simulink subsystem "PvtSubSys_LATC"  (R2020b)
settings: Solver=VariableStepAuto  StartTime=0.0  StopTime=10.0  RelTol=1e-3
values from neighbouring files (symbols this model uses):
  P_Global_CharSpd_ms : value not decoded    [PubParsGlobal.sldd]
  P_Global_SteeringAngleRatio : value not decoded    [PubParsGlobal.sldd]
  P_Global_WheelBase_m : value not decoded    [PubParsGlobal.sldd]
  P_LCS_A0_Limit = 0.25    [LATC.sldd]    (also in LCS_v05.sldd)
  P_LCS_A1_Limit = 0.002    [LATC.sldd]    (also in LCS_v05.sldd)
  P_LCS_communicationTest = 1.0    [LATC.sldd]    (also in LCS_v05.sldd)
  P_LCS_Current_Offset_Test_SW = 0.0    [LATC.sldd]
  P_LCS_Current_Offset_Test_Value = 0.0    [LATC.sldd]
  P_LCS_Curvature_bp : value not decoded    [LATC.sldd]
  P_LCS_CycleTime = 0.4 0.4 0.4 0.4 0.4 0.4 0.4 0.4 0.4 0.6 0.6 0.6 0.6 0.6 0.6 0.6 0.4 0.4 0.4 0.4 0.4 0.4 0.4 0.4 0.4 0.6 0.6 0.6 0.6 0.6 0.6 0.6 0.4 0.4 0.4 0.4 0.4 0.4 0.4 0.4 0.4 0.6 0.6 0.6 0.6 0.6 0.6 0.6 0.4 0.4 0.4 0.4 0.4 0.4 0.4 0.4 0.4 0.6 0.6 0.6 0.6 0.6 0.6 0.6 0.4 0.4 0.4 0.4 0.4 0.4 0.4 0.4 0.4 0.6 0.6 0.6 0.6 0.6 0.6 0.6 0.4 0.4 0.4 0.4 0.4 0.4 0.4 0.4 0.4 0.6 0.6 0.6 0.6 0.6 0.6 0.6 0.4 0.4 0.4 0.4    [LATC.sldd]
  P_LCS_ESS_AngleSlope_Limit = 2.9    [LATC.sldd]    (also in LCS_v05.sldd)
  P_LCS_IN_Offset_Test_SW = 0.0    [LATC.sldd]    (also in LCS_v05.sldd)
  P_LCS_IN_Offset_Test_Value = 0.0    [LATC.sldd]    (also in LCS_v05.sldd)
  P_LCS_LATC_CurOffsetVehicleSpdLimitValue_degs = 7.0    [LATC.sldd]
  P_LCS_LATC_Du_Max = 20.0    [LATC.sldd]
  P_LCS_LATC_ELKAngleSlope_ratio : value not decoded    [LATC.sldd]
  P_LCS_LATC_ELKMaxLatAcc_ms2 : value not decoded    [LATC.sldd]
  P_LCS_LATC_ESSAngleSlope_ratio : value not decoded    [LATC.sldd]
  P_LCS_LATC_ESSMaxLatAcc_ms2 : value not decoded    [LATC.sldd]
  P_LCS_LATC_LCAngleSlope_ratio : value not decoded    [LATC.sldd]
  P_LCS_LATC_LCCancleMaxLatAcc_ms2 : value not decoded    [LATC.sldd]
  P_LCS_LATC_LCEcoAngleSlope_ratio : value not decoded    [LATC.sldd]
  P_LCS_LATC_LCEcoMaxLatAcc_ms2 : value not decoded    [LATC.sldd]
  P_LCS_LATC_LCKAngleSlope_ratio : value not decoded    [LATC.sldd]
  P_LCS_LATC_LCKIEAngleSlope_ratio : value not decoded    [LATC.sldd]
  P_LCS_LATC_LCKIEMaxLatAcc_ms2 : value not decoded    [LATC.sldd]
  P_LCS_LATC_LCKMaxLatAcc_ms2 : value not decoded    [LATC.sldd]
  P_LCS_LATC_LCNormalAngleSlope_ratio : value not decoded    [LATC.sldd]
  P_LCS_LATC_LCNormalMaxLatAcc_ms2 : value not decoded    [LATC.sldd]
  P_LCS_LATC_LCSportAngleSlope_ratio : value not decoded    [LATC.sldd]
  P_LCS_LATC_LCSportMaxLatAcc_ms2 : value not decoded    [LATC.sldd]
  P_LCS_LATC_LKAAngleSlope_ratio : value not decoded    [LATC.sldd]
  P_LCS_LATC_LKAMaxLatAcc_ms2 : value not decoded    [LATC.sldd]
  P_LCS_LATC_MatrixQ1_st = 0.8 0.8 1.2 1.4 1.4 1.4 2.0 2.2 2.2 2.2 2.2 2.2 2.2 2.2 2.2 2.2 0.8 0.8 1.2 1.4 1.4 1.4 2.0 2.2 2.2 2.2 2.2 2.2 2.2 2.2 2.2 2.2 0.8 0.8 1.2 1.4 1.4 1.4 2.0 2.2 2.2 2.2 2.2 2.2 2.2 2.2 2.2 2.2 0.8 0.8 1.2 1.4 1.4 1.4 2.0 2.2 2.2 2.2 2.2 2.2 2.2 2.2 2.2 2.2 0.8 0.8 1.2 1.4 1.4 1.4 2.0 2.2 2.2 2.2 2.2 2.2 2.2 2.2 2.2 2.2 0.8 0.8 1.2 1.4 1.4 1.4 2.0 2.2 2.2 2.2 2.2 2.2 2.2 2.2 2.2 2.2 0.8 0.8 1.2 1.4    [LATC.sldd]
  P_LCS_LATC_MatrixQ3_st = 20.0 20.0 20.0 20.0 20.0 15.0 15.0 15.0 15.0 15.0 15.0 15.0 15.0 13.0 13.0 13.0 20.0 20.0 20.0 20.0 20.0 15.0 15.0 15.0 15.0 15.0 15.0 15.0 15.0 13.0 13.0 13.0 20.0 20.0 20.0 20.0 20.0 15.0 15.0 15.0 15.0 15.0 15.0 15.0 15.0 13.0 13.0 13.0 20.0 20.0 20.0 20.0 20.0 15.0 15.0 15.0 15.0 15.0 15.0 15.0 15.0 13.0 13.0 13.0 20.0 20.0 20.0 20.0 20.0 15.0 15.0 15.0 15.0 15.0 15.0 15.0 15.0 13.0 13.0 13.0    [LATC.sldd]
  P_LCS_LATC_MatrixR_st = 10.0 10.0 10.0 10.0 10.0 10.0 10.0 15.0 15.0 15.0 15.0 15.0 15.0 15.0 15.0 15.0 10.0 10.0 10.0 10.0 10.0 10.0 10.0 15.0 15.0 15.0 15.0 15.0 15.0 15.0 15.0 15.0 10.0 10.0 10.0 10.0 10.0 10.0 10.0 15.0 15.0 15.0 15.0 15.0 15.0 15.0 15.0 15.0 10.0 10.0 10.0 10.0 10.0 10.0 10.0 15.0 15.0 15.0 15.0 15.0 15.0 15.0 15.0 15.0 10.0 10.0 10.0 10.0 10.0 10.0 10.0 15.0 15.0 15.0 15.0 15.0 15.0 15.0 15.0 15.0    [LATC.sldd]
  P_LCS_LATC_Max_LatAcc = 4.0    [LATC.sldd]
  P_LCS_LATC_Max_Phi = 15.0    [LATC.sldd]
  P_LCS_LATC_Max_y = 0.5    [LATC.sldd]
  P_LCS_LATC_MPC_SW = 0.0    [LATC.sldd]
  P_LCS_LATC_PreView_SW = 1.0    [LATC.sldd]
  P_LCS_LATC_SoftConstWeight = 1.0    [LATC.sldd]
  P_LCS_LATC_StateActivAngleSlopeLimit_ratio : value not decoded    [LATC.sldd]
  P_LCS_LATC_StateActiveFlg_TabX_st : value not decoded    [LATC.sldd]
  P_LCS_LATC_StateActiveHoldTime_TabY_st : value not decoded    [LATC.sldd]
  P_LCS_LATC_StateHoldTime_st = 250.0    [LATC.sldd]
  P_LCS_LATC_TarAngleFliterWindowSize = 5.0    [LATC.sldd]
  P_LCS_LATC_TarAngleLP_Time = 0.02    [LATC.sldd]
  P_LCS_LATC_U_Max = 90.0    [LATC.sldd]
  P_LCS_LCK_AngleSlope_Limit = 1.4    [LATC.sldd]
  P_LCS_LineVaildSW = 0.0    [LATC.sldd]
  P_LCS_Lookahead_Distance : value not decoded    [LATC.sldd]
  P_LCS_Lookahead_DistanceFac : value not decoded    [LATC.sldd]
  P_LCS_PLAN_CurvePreView_s = 0.3    [LATC.sldd]
  P_LCS_PLAN_CurvePreview_TabX_m : value not decoded    [LATC.sldd]
  P_LCS_PLAN_CurvePreViewFilterTime_s = 0.1    [LATC.sldd]
  P_LCS_PLAN_ELKAyDtLimit_Tab_ms3 = 1.0 1.0 1.0 1.0 1.0 1.0 1.0 1.0 1.0 1.0 1.0 1.0 1.0 1.0 1.0 1.0 1.0 1.0 1.0 1.0 1.0 1.0 1.0 1.0 1.0 1.0 1.0 1.0 1.0 1.0 1.0 1.0 1.0 1.0 1.0 1.0 1.0 1.0 1.0 1.0 1.0 1.0 1.0 1.0 1.0 1.0 1.0 1.0 1.0 1.0 1.0 1.0 1.0 1.0 1.0 1.0 1.0 1.0 1.0 1.0 1.0 1.0 1.0 1.0 1.0 1.0 1.0 1.0 1.0 1.0 1.0 1.0 1.0 1.0 1.0 1.0 1.0 1.0 1.0 1.0 1.0 1.0 1.0 1.0 1.0 1.0 1.0 1.0 1.0 1.0 1.0 1.0 1.0 1.0 1.0 1.0 1.0 1.0 1.0 1.0    [LATC.sldd]
  P_LCS_PLAN_ESSAyDtLimit_Tab_ms3 = 1.0 1.0 1.0 1.0 1.0 1.0 1.0 1.0 1.0 1.0 1.0 1.0 1.0 1.0 1.0 1.0 1.0 1.0 1.0 1.0 1.0 1.0 1.0 1.0 1.0 1.0 1.0 1.0 1.0 1.0 1.0 1.0 1.0 1.0 1.0 1.0 1.0 1.0 1.0 1.0 1.0 1.0 1.0 1.0 1.0 1.0 1.0 1.0 1.0 1.0 1.0 1.0 1.0 1.0 1.0 1.0 1.0 1.0 1.0 1.0 1.0 1.0 1.0 1.0 1.0 1.0 1.0 1.0 1.0 1.0 1.0 1.0 1.0 1.0 1.0 1.0 1.0 1.0 1.0 1.0 1.0 1.0 1.0 1.0 1.0 1.0 1.0 1.0 1.0 1.0 1.0 1.0 1.0 1.0 1.0 1.0 1.0 1.0 1.0 1.0    [LATC.sldd]
  P_LCS_PLAN_LCCancleAyDtLimit_Tab_ms3 = 1.0 1.0 1.0 1.0 1.0 1.0 1.0 1.0 1.0 1.0 1.0 1.0 1.0 1.0 1.0 1.0 1.0 1.0 1.0 1.0 1.0 1.0 1.0 1.0 1.0 1.0 1.0 1.0 1.0 1.0 1.0 1.0 1.0 1.0 1.0 1.0 1.0 1.0 1.0 1.0 1.0 1.0 1.0 1.0 1.0 1.0 1.0 1.0 1.0 1.0 1.0 1.0 1.0 1.0 1.0 1.0 1.0 1.0 1.0 1.0 1.0 1.0 1.0 1.0 1.0 1.0 1.0 1.0 1.0 1.0 1.0 1.0 1.0 1.0 1.0 1.0 1.0 1.0 1.0 1.0 1.0 1.0 1.0 1.0 1.0 1.0 1.0 1.0 1.0 1.0 1.0 1.0 1.0 1.0 1.0 1.0 1.0 1.0 1.0 1.0    [LATC.sldd]
  P_LCS_PLAN_LCEcoAyDtLimit_Tab_ms3 = 1.0 1.0 1.0 1.0 1.0 1.0 1.0 1.0 1.0 1.0 1.0 1.0 1.0 1.0 1.0 1.0 1.0 1.0 1.0 1.0 1.0 1.0 1.0 1.0 1.0 1.0 1.0 1.0 1.0 1.0 1.0 1.0 1.0 1.0 1.0 1.0 1.0 1.0 1.0 1.0 1.0 1.0 1.0 1.0 1.0 1.0 1.0 1.0 1.0 1.0 1.0 1.0 1.0 1.0 1.0 1.0 1.0 1.0 1.0 1.0 1.0 1.0 1.0 1.0 1.0 1.0 1.0 1.0 1.0 1.0 1.0 1.0 1.0 1.0 1.0 1.0 1.0 1.0 1.0 1.0 1.0 1.0 1.0 1.0 1.0 1.0 1.0 1.0 1.0 1.0 1.0 1.0 1.0 1.0 1.0 1.0 1.0 1.0 1.0 1.0    [LATC.sldd]
  P_LCS_PLAN_LCKAyDtLimit_Tab_ms3 = 1.5 1.5 1.5 1.5 1.5 1.5 1.5 1.5 1.5 1.5 1.5 1.5 1.5 1.5 1.5 1.5 1.5 1.5 1.5 1.5 1.5 1.5 1.5 1.5 1.5 1.5 1.5 1.5 1.5 1.5 1.5 1.5 1.5 1.5 1.5 1.5 1.5 1.5 1.5 1.5 1.5 1.5 1.5 1.5 1.5 1.5 1.5 1.5 1.5 1.5 1.5 1.5 1.5 1.5 1.5 1.5 1.5 1.5 1.5 1.5 1.5 1.5 1.5 1.5 1.5 1.5 1.5 1.5 1.5 1.5 1.5 1.5 1.5 1.5 1.5 1.5 1.5 1.5 1.5 1.5 1.5 1.5 1.5 1.5 1.5 1.5 1.5 1.5 1.5 1.5 1.5 1.5 1.5 1.5 1.5 1.5 1.5 1.5 1.5 1.5    [LATC.sldd]
  P_LCS_PLAN_LCKIEAyDtLimit_Tab_ms3 = 1.0 1.0 1.0 1.0 1.0 1.0 1.0 1.0 1.0 1.0 1.0 1.0 1.0 1.0 1.0 1.0 1.0 1.0 1.0 1.0 1.0 1.0 1.0 1.0 1.0 1.0 1.0 1.0 1.0 1.0 1.0 1.0 1.0 1.0 1.0 1.0 1.0 1.0 1.0 1.0 1.0 1.0 1.0 1.0 1.0 1.0 1.0 1.0 1.0 1.0 1.0 1.0 1.0 1.0 1.0 1.0 1.0 1.0 1.0 1.0 1.0 1.0 1.0 1.0 1.0 1.0 1.0 1.0 1.0 1.0 1.0 1.0 1.0 1.0 1.0 1.0 1.0 1.0 1.0 1.0 1.0 1.0 1.0 1.0 1.0 1.0 1.0 1.0 1.0 1.0 1.0 1.0 1.0 1.0 1.0 1.0 1.0 1.0 1.0 1.0    [LATC.sldd]
  P_LCS_PLAN_LCNormalAyDtLimit_Tab_ms3 = 1.0 1.0 1.0 1.0 1.0 1.0 1.0 1.0 1.0 1.0 1.0 1.0 1.0 1.0 1.0 1.0 1.0 1.0 1.0 1.0 1.0 1.0 1.0 1.0 1.0 1.0 1.0 1.0 1.0 1.0 1.0 1.0 1.0 1.0 1.0 1.0 1.0 1.0 1.0 1.0 1.0 1.0 1.0 1.0 1.0 1.0 1.0 1.0 1.0 1.0 1.0 1.0 1.0 1.0 1.0 1.0 1.0 1.0 1.0 1.0 1.0 1.0 1.0 1.0 1.0 1.0 1.0 1.0 1.0 1.0 1.0 1.0 1.0 1.0 1.0 1.0 1.0 1.0 1.0 1.0 1.0 1.0 1.0 1.0 1.0 1.0 1.0 1.0 1.0 1.0 1.0 1.0 1.0 1.0 1.0 1.0 1.0 1.0 1.0 1.0    [LATC.sldd]
  P_LCS_PLAN_LCSportAyDtLimit_Tab_ms3 = 1.0 1.0 1.0 1.0 1.0 1.0 1.0 1.0 1.0 1.0 1.0 1.0 1.0 1.0 1.0 1.0 1.0 1.0 1.0 1.0 1.0 1.0 1.0 1.0 1.0 1.0 1.0 1.0 1.0 1.0 1.0 1.0 1.0 1.0 1.0 1.0 1.0 1.0 1.0 1.0 1.0 1.0 1.0 1.0 1.0 1.0 1.0 1.0 1.0 1.0 1.0 1.0 1.0 1.0 1.0 1.0 1.0 1.0 1.0 1.0 1.0 1.0 1.0 1.0 1.0 1.0 1.0 1.0 1.0 1.0 1.0 1.0 1.0 1.0 1.0 1.0 1.0 1.0 1.0 1.0 1.0 1.0 1.0 1.0 1.0 1.0 1.0 1.0 1.0 1.0 1.0 1.0 1.0 1.0 1.0 1.0 1.0 1.0 1.0 1.0    [LATC.sldd]
  P_LCS_PLAN_LKAAyDtLimit_Tab_ms3 = 1.0 1.0 1.0 1.0 1.0 1.0 1.0 1.0 1.0 1.0 1.0 1.0 1.0 1.0 1.0 1.0 1.0 1.0 1.0 1.0 1.0 1.0 1.0 1.0 1.0 1.0 1.0 1.0 1.0 1.0 1.0 1.0 1.0 1.0 1.0 1.0 1.0 1.0 1.0 1.0 1.0 1.0 1.0 1.0 1.0 1.0 1.0 1.0 1.0 1.0 1.0 1.0 1.0 1.0 1.0 1.0 1.0 1.0 1.0 1.0 1.0 1.0 1.0 1.0 1.0 1.0 1.0 1.0 1.0 1.0 1.0 1.0 1.0 1.0 1.0 1.0 1.0 1.0 1.0 1.0 1.0 1.0 1.0 1.0 1.0 1.0 1.0 1.0 1.0 1.0 1.0 1.0 1.0 1.0 1.0 1.0 1.0 1.0 1.0 1.0    [LATC.sldd]
  P_LCS_PLAN_MinPlanDis_m : value not decoded    [LATC.sldd]
  P_LCS_PLAN_PreCurMinDisFac_ratio : value not decoded    [LATC.sldd]
  P_LCS_PLAN_PreDisCurve_TabX_m : value not decoded    [LATC.sldd]
  P_LCS_PLAN_StateActiv_AyDtLimit_ms3 : value not decoded    [LATC.sldd]
  P_LCS_PLAN_VehicleSpd_TabX_kph : value not decoded    [LATC.sldd]
  P_LCS_PLAN_VehicleSpd_TabY_Kph : value not decoded    [LATC.sldd]
  P_LCS_Trq_Switch = 0.0    [LATC.sldd]    (also in LCS_v05.sldd)
  P_LCS_VehicleSpd_TabX_Kph : value not decoded    [LATC.sldd]
undefined symbols (not defined in the file or in its folder): HWP_AngCmdReqVal, HWP_AngCmdReqValVld, HWP_FuncTrqCmdReqFlag, HWP_ReqCtrlEPS, HWP_ReqCtrlEPSVld, HWP_TrqOvlCmdReqValue, HWP_WorkReq, HWP_WorkReqVld
libraries: simulink x4, dspbuff3 x2
(part 5 of 8)

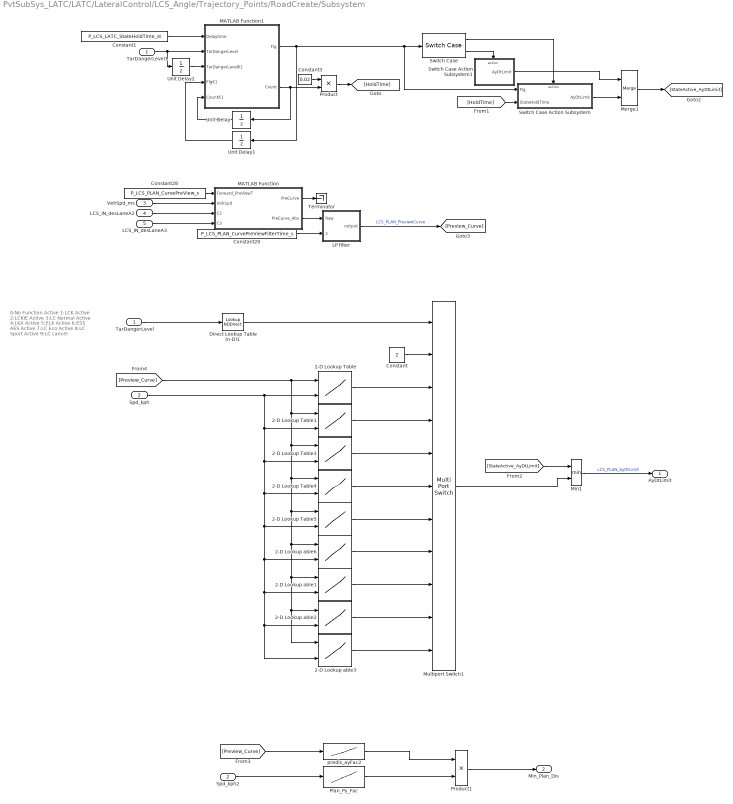
== system PvtSubSys_LATC/LATC/LateralControl/LCS_Angle/Trajectory_Points/RoadCreate/Subsystem ==
  note: 0:No Function Active
      | 1:LCK Active
      | 2:LCKIE Active
      | 3:LC Normal Active
      | 4:LKA Active
      | 5:ELK Active
      | 6:ESS AES Active
      | 7:LC Eco Active
      | 8:LC Sport Active
      | 9:LC cancel
  TarDangerLevel : Inport
  Spd_kph : Inport  Port=2
  VehSpd_ms : Inport  Port=3
  LCS_IN_desLaneA2 : Inport  Port=4
  LCS_IN_desLaneA3 : Inport  Port=5
  2-D Lookup Table : Lookup_n-D  BreakpointsForDimension1=P_LCS_PLAN_PreDisCurve_TabX_m  BreakpointsForDimension2=P_LCS_PLAN_VehicleSpd_TabY_Kph  Table=P_LCS_PLAN_LCKAyDtLimit_Tab_ms3  InternalRulePriority=Speed  RndMeth=Simplest  InputSameDT=on
      settings: InputPortMap=u0,u1
  2-D Lookup Table1 : Lookup_n-D  BreakpointsForDimension1=P_LCS_PLAN_PreDisCurve_TabX_m  BreakpointsForDimension2=P_LCS_PLAN_VehicleSpd_TabY_Kph  Table=P_LCS_PLAN_LCKIEAyDtLimit_Tab_ms3  InternalRulePriority=Speed  RndMeth=Simplest  InputSameDT=on
      settings: InputPortMap=u0,u1
  2-D Lookup Table3 : Lookup_n-D  BreakpointsForDimension1=P_LCS_PLAN_PreDisCurve_TabX_m  BreakpointsForDimension2=P_LCS_PLAN_VehicleSpd_TabY_Kph  Table=P_LCS_PLAN_LCNormalAyDtLimit_Tab_ms3  InternalRulePriority=Speed  RndMeth=Simplest  InputSameDT=on
      settings: InputPortMap=u0,u1
  2-D Lookup Table4 : Lookup_n-D  BreakpointsForDimension1=P_LCS_PLAN_PreDisCurve_TabX_m  BreakpointsForDimension2=P_LCS_PLAN_VehicleSpd_TabY_Kph  Table=P_LCS_PLAN_LKAAyDtLimit_Tab_ms3  InternalRulePriority=Speed  RndMeth=Simplest  InputSameDT=on
      settings: InputPortMap=u0,u1
  2-D Lookup Table5 : Lookup_n-D  BreakpointsForDimension1=P_LCS_PLAN_PreDisCurve_TabX_m  BreakpointsForDimension2=P_LCS_PLAN_VehicleSpd_TabY_Kph  Table=P_LCS_PLAN_ELKAyDtLimit_Tab_ms3  InternalRulePriority=Speed  RndMeth=Simplest  InputSameDT=on
      settings: InputPortMap=u0,u1
  2-D Lookup able1 : Lookup_n-D  BreakpointsForDimension1=P_LCS_PLAN_PreDisCurve_TabX_m  BreakpointsForDimension2=P_LCS_PLAN_VehicleSpd_TabY_Kph  Table=P_LCS_PLAN_LCEcoAyDtLimit_Tab_ms3  InternalRulePriority=Speed  RndMeth=Simplest  InputSameDT=on
      settings: InputPortMap=u0,u1
  2-D Lookup able2 : Lookup_n-D  BreakpointsForDimension1=P_LCS_PLAN_PreDisCurve_TabX_m  BreakpointsForDimension2=P_LCS_PLAN_VehicleSpd_TabY_Kph  Table=P_LCS_PLAN_LCSportAyDtLimit_Tab_ms3  InternalRulePriority=Speed  RndMeth=Simplest  InputSameDT=on
      settings: InputPortMap=u0,u1
  2-D Lookup able3 : Lookup_n-D  BreakpointsForDimension1=P_LCS_PLAN_PreDisCurve_TabX_m  BreakpointsForDimension2=P_LCS_PLAN_VehicleSpd_TabY_Kph  Table=P_LCS_PLAN_LCCancleAyDtLimit_Tab_ms3  InternalRulePriority=Speed  RndMeth=Simplest  InputSameDT=on
      settings: InputPortMap=u0,u1
  2-D Lookup able6 : Lookup_n-D  BreakpointsForDimension1=P_LCS_PLAN_PreDisCurve_TabX_m  BreakpointsForDimension2=P_LCS_PLAN_VehicleSpd_TabY_Kph  Table=P_LCS_PLAN_ESSAyDtLimit_Tab_ms3  InternalRulePriority=Speed  RndMeth=Simplest  InputSameDT=on
      settings: InputPortMap=u0,u1
  Constant : Constant  Value=2  OutDataTypeStr=single
  Constant1 : Constant  Value=P_LCS_LATC_StateHoldTime_st  OutDataTypeStr=uint16
  Constant20 : Constant  Value=P_LCS_PLAN_CurvePreViewFilterTime_s  OutDataTypeStr=single
  Constant28 : Constant  Value=P_LCS_PLAN_CurvePreView_s  OutDataTypeStr=single
  Constant3 : Constant  Value=0.02
  Direct Lookup Table (n-D)1 : LookupNDDirect  NumberOfTableDimensions=1  Table=[0 1 2 3 4 5 6 7 8 9]  TableDataTypeStr=uint8
  LP filter : Subsystem
  MATLAB Function : MATLAB Function  TreatAsAtomicUnit=on
  MATLAB Function1 : MATLAB Function  TreatAsAtomicUnit=on
  Merge1 : Merge
  Min1 : MinMax  Inputs=2
  Multiport Switch1 : MultiPortSwitch  DataPortOrder=Zero-based contiguous  Inputs=10  zeroidx=on
  Plan_Py_Fac : Lookup_n-D  NumberOfTableDimensions=1  BreakpointsForDimension1=P_LCS_PLAN_VehicleSpd_TabX_kph  Table=P_LCS_PLAN_MinPlanDis_m  ExtrapMethod=Clip  UseLastTableValue=on  InternalRulePriority=Speed  RndMeth=Simplest  InputSameDT=on
  Product : Product
  Product1 : Product
  Spd_kph2 : InportShadow  Port=2
  Switch Case : SwitchCase  CaseConditions={[1]}
  Switch Case Action Subsystem : Subsystem  TreatAsAtomicUnit=on
  Switch Case Action Subsystem1 : Subsystem  TreatAsAtomicUnit=on
  TarDangerLevel1 : InportShadow
  Terminator : Terminator
  Unit Delay : UnitDelay  SampleTime=-1  HasFrameUpgradeWarning=on
  Unit Delay1 : UnitDelay  SampleTime=-1  HasFrameUpgradeWarning=on
  Unit Delay2 : UnitDelay  SampleTime=-1  HasFrameUpgradeWarning=on
  predis_ayFac2 : Lookup_n-D  NumberOfTableDimensions=1  BreakpointsForDimension1=P_LCS_PLAN_CurvePreview_TabX_m  Table=P_LCS_PLAN_PreCurMinDisFac_ratio  ExtrapMethod=Clip  UseLastTableValue=on  InternalRulePriority=Speed  RndMeth=Simplest  InputSameDT=on
  AyDtLimit : Outport  OutDataTypeStr=single
  Min_Plan_Dis : Outport  Port=2  OutDataTypeStr=single
  wires:
  2-D Lookup Table/1 -> Multiport Switch1/3
  Multiport Switch1/1 -> Min1/2
  [StateActive_AyDtLimit] -> Min1/1
  Merge1/1 -> [StateActive_AyDtLimit]
  Switch Case Action Subsystem1/1(AyDtLimit) -> Merge1/1
  Switch Case Action Subsystem/1(AyDtLimit) -> Merge1/2
  Product/1 -> [HoldTime]
  [HoldTime] -> Switch Case Action Subsystem/2(StateHoldTime)
  Constant3/1 -> Product/1
  Switch Case/2 -> Switch Case Action Subsystem1/Action
  MATLAB Function1/2(Count) -> Unit Delay/1, Product/2
  Switch Case/1 -> Switch Case Action Subsystem/Action
  MATLAB Function1/1(Flg) -> Switch Case/1, Switch Case Action Subsystem/1(Flg), Unit Delay1/1
  Constant1/1 -> MATLAB Function1/1(Delaytime)
  Unit Delay2/1 -> MATLAB Function1/3(TarDangerLevelK1)
  TarDangerLevel1/1 -> MATLAB Function1/2(TarDangerLevel), Unit Delay2/1
  Unit Delay1/1 -> MATLAB Function1/4(FlgK1)
  Unit Delay/1 -> MATLAB Function1/5(CountK1)
  2-D Lookup Table5/1 -> Multiport Switch1/7
  2-D Lookup Table3/1 -> Multiport Switch1/5
  2-D Lookup Table1/1 -> Multiport Switch1/4
  Constant/1 -> Multiport Switch1/2
  Constant28/1 -> MATLAB Function/1(Forward_PreViewT)
  LP filter/1(output) -> [Preview_Curve]  "LCS_PLAN_PreviewCurve"
  Constant20/1 -> LP filter/2(TorqFilterTime)
  LCS_IN_desLaneA3/1 -> MATLAB Function/4(C3)
  LCS_IN_desLaneA2/1 -> MATLAB Function/3(C2)
  VehSpd_ms/1 -> MATLAB Function/2(VehSpd)
  Min1/1 -> AyDtLimit/1  "LCS_PLAN_AyDtLimit"
  TarDangerLevel/1 -> Direct Lookup Table (n-D)1/1
  Direct Lookup Table (n-D)1/1 -> Multiport Switch1/1
  Plan_Py_Fac/1 -> Product1/2
  Spd_kph2/1 -> Plan_Py_Fac/1
  [Preview_Curve] -> predis_ayFac2/1
  Product1/1 -> Min_Plan_Dis/1
  predis_ayFac2/1 -> Product1/1
  MATLAB Function/2(PreCurve_Abs) -> LP filter/1(Raw)
  MATLAB Function/1(PreCurve) -> Terminator/1
  [Preview_Curve] -> 2-D Lookup able3/1, 2-D Lookup able2/1, 2-D Lookup able1/1, 2-D Lookup able6/1, 2-D Lookup Table5/1, 2-D Lookup Table4/1, 2-D Lookup Table3/1, 2-D Lookup Table1/1, 2-D Lookup Table/1
  Spd_kph/1 -> 2-D Lookup Table/2, 2-D Lookup Table1/2, 2-D Lookup Table3/2, 2-D Lookup Table4/2, 2-D Lookup able3/2, 2-D Lookup able2/2, 2-D Lookup able1/2, 2-D Lookup able6/2, 2-D Lookup Table5/2
  2-D Lookup Table4/1 -> Multiport Switch1/6
  2-D Lookup able6/1 -> Multiport Switch1/8
  2-D Lookup able1/1 -> Multiport Switch1/9
  2-D Lookup able2/1 -> Multiport Switch1/10
  2-D Lookup able3/1 -> Multiport Switch1/11

== system PvtSubSys_LATC/LATC/LateralControl/LCS_Angle/Controller/TargetAngleCalc/MedianLowPass_Filter/LP ==
  Raw : Inport
  Constant1 : Constant  Value=P_LCS_LATC_TarAngleLP_Time  OutDataTypeStr=single
  Constant3 : Constant  Value=0.02  OutDataTypeStr=single
  Product7 : Product  Inputs=*/  RndMeth=Zero
  Product8 : Product  RndMeth=Zero
  Sum14 : Sum
  Sum9 : Sum  Inputs=+-
  Unit Delay : UnitDelay  SampleTime=-1  HasFrameUpgradeWarning=on
  Out : Outport
  wires:
  Constant1/1 -> Product7/2
  Constant3/1 -> Product7/1
  Sum9/1 -> Product8/2
  Sum14/1 -> Out/1, Unit Delay/1
  Unit Delay/1 -> Sum14/2, Sum9/2
  Raw/1 -> Sum9/1
  Product8/1 -> Sum14/1
  Product7/1 -> Product8/1

== system PvtSubSys_LATC/LATC/LateralControl/LCS_Angle/Controller/TargetAngleCalc/MedianLowPass_Filter/Median_Filter ==
  In : Inport
  Add : Sum  Inputs=+-
  Constant : Constant  Value=2  OutDataTypeStr=single
  Constant11 : Constant  Value=P_LCS_LATC_TarAngleFliterWindowSize  OutDataTypeStr=single
  Delay Line : dspbuff3/Delay Line  siz=P_LCS_LATC_TarAngleFliterWindowSize  ic=0  directfeed=off  enable_output=off  hold_output=off  OutputFrames=off
      settings: SourceProductBaseCode=DS
  Divide1 : Product  Inputs=*/
  Max of Elements1 : MinMax  Function=max
  MinMax2 : MinMax
  Minus1 : Sum  Inputs=--+
  Sum of Elements1 : Sum  Inputs=+
  Out : Outport
  wires:
  Max of Elements1/1 -> Minus1/2
  Divide1/1 -> Out/1
  Minus1/1 -> Divide1/1
  In/1 -> Delay Line/1
  MinMax2/1 -> Minus1/1
  Sum of Elements1/1 -> Minus1/3
  Delay Line/1 -> Max of Elements1/1, MinMax2/1, Sum of Elements1/1
  Constant11/1 -> Add/1
  Add/1 -> Divide1/2
  Constant/1 -> Add/2

== system PvtSubSys_LATC/LATC/LateralControl/LCS_Angle/Controller/TargetAngleCalc/MedianLowPass_Filter1/LP ==
  Raw : Inport
  Constant1 : Constant  Value=0.02  OutDataTypeStr=single
  Constant3 : Constant  Value=0.02  OutDataTypeStr=single
  Product7 : Product  Inputs=*/  RndMeth=Zero
  Product8 : Product  RndMeth=Zero
  Sum14 : Sum
  Sum9 : Sum  Inputs=+-
  Unit Delay : UnitDelay  SampleTime=-1  HasFrameUpgradeWarning=on
  Out : Outport
  wires:
  Constant1/1 -> Product7/2
  Constant3/1 -> Product7/1
  Sum9/1 -> Product8/2
  Sum14/1 -> Out/1, Unit Delay/1
  Unit Delay/1 -> Sum14/2, Sum9/2
  Raw/1 -> Sum9/1
  Product8/1 -> Sum14/1
  Product7/1 -> Product8/1

== system PvtSubSys_LATC/LATC/LateralControl/LCS_Angle/Controller/TargetAngleCalc/MedianLowPass_Filter1/Median_Filter ==
  In : Inport
  Add : Sum  Inputs=+-
  Constant : Constant  Value=2  OutDataTypeStr=single
  Constant11 : Constant  Value=P_LCS_LATC_TarAngleFliterWindowSize  OutDataTypeStr=single
  Delay Line : dspbuff3/Delay Line  siz=P_LCS_LATC_TarAngleFliterWindowSize  ic=0  directfeed=off  enable_output=off  hold_output=off  OutputFrames=off
      settings: SourceProductBaseCode=DS
  Divide1 : Product  Inputs=*/
  Max of Elements1 : MinMax  Function=max
  MinMax2 : MinMax
  Minus1 : Sum  Inputs=--+
  Sum of Elements1 : Sum  Inputs=+
  Out : Outport
  wires:
  Max of Elements1/1 -> Minus1/2
  Divide1/1 -> Out/1
  Minus1/1 -> Divide1/1
  In/1 -> Delay Line/1
  MinMax2/1 -> Minus1/1
  Sum of Elements1/1 -> Minus1/3
  Delay Line/1 -> Max of Elements1/1, MinMax2/1, Sum of Elements1/1
  Constant11/1 -> Add/1
  Add/1 -> Divide1/2
  Constant/1 -> Add/2

== system PvtSubSys_LATC/LATC/LateralControl/LCS_Angle/Controller/TargetAngleCalc/SteerAngSlopeCalc/Switch Case Action Subsystem ==
  Flg : Inport
  StateHoldTime : Inport  Port=2
  Action Port : ActionPort
  LC_start_slope : Lookup_n-D  BreakpointsForDimension1=P_LCS_LATC_StateActiveFlg_TabX_st  BreakpointsForDimension2=P_LCS_LATC_StateActiveHoldTime_TabY_st  Table=P_LCS_LATC_StateActivAngleSlopeLimit_ratio  ExtrapMethod=Clip  UseLastTableValue=on  InternalRulePriority=Speed  OutDataTypeStr=single  RndMeth=Simplest
      settings: InputPortMap=u0,u1
  Out1 : Outport
  wires:
  StateHoldTime/1 -> LC_start_slope/2
  LC_start_slope/1 -> Out1/1
  Flg/1 -> LC_start_slope/1

== system PvtSubSys_LATC/LATC/LateralControl/LCS_Angle/Controller/TargetAngleCalc/SteerAngSlopeCalc/Switch Case Action Subsystem1 ==
  Action Port : ActionPort
  Constant : Constant  Value=100  OutDataTypeStr=single
  Out1 : Outport
  wires:
  Constant/1 -> Out1/1

== system PvtSubSys_LATC/LATC/LateralControl/LCS_Angle/Trajectory_Points/RoadCreate/Subsystem/LP filter ==
  Raw : Inport
  TorqFilterTime : Inport  Port=2
  Product1 : Product  RndMeth=Zero
  Product4 : Product  Inputs=*/  RndMeth=Zero
  Sum4 : Sum  Inputs=+-
  Sum5 : Sum
  Unit Delay : UnitDelay  SampleTime=-1  HasFrameUpgradeWarning=on
  Weight/N3 : Constant  Value=0.02  OutDataTypeStr=single
  output : Outport
  wires:
  TorqFilterTime/1 -> Product4/2
  Product4/1 -> Product1/1
  Weight/N3/1 -> Product4/1
  Raw/1 -> Sum4/1
  Product1/1 -> Sum5/1
  Sum4/1 -> Product1/2
  Unit Delay/1 -> Sum4/2, Sum5/2
  Sum5/1 -> Unit Delay/1, output/1

== system PvtSubSys_LATC/LATC/LateralControl/LCS_Angle/Trajectory_Points/RoadCreate/Subsystem/Switch Case Action Subsystem ==
  Flg : Inport
  StateHoldTime : Inport  Port=2
  Action Port : ActionPort
  ActiveAyDtLimit_TBL : Lookup_n-D  BreakpointsForDimension1=P_LCS_LATC_StateActiveFlg_TabX_st  BreakpointsForDimension2=P_LCS_LATC_StateActiveHoldTime_TabY_st  Table=P_LCS_PLAN_StateActiv_AyDtLimit_ms3  ExtrapMethod=Clip  UseLastTableValue=on  InternalRulePriority=Speed  OutDataTypeStr=single  RndMeth=Simplest
      settings: InputPortMap=u0,u1
  AyDtLimit : Outport
  wires:
  ActiveAyDtLimit_TBL/1 -> AyDtLimit/1
  Flg/1 -> ActiveAyDtLimit_TBL/1
  StateHoldTime/1 -> ActiveAyDtLimit_TBL/2

== system PvtSubSys_LATC/LATC/LateralControl/LCS_Angle/Trajectory_Points/RoadCreate/Subsystem/Switch Case Action Subsystem1 ==
  Action Port : ActionPort
  Constant1 : Constant  Value=100  OutDataTypeStr=single
  AyDtLimit : Outport
  wires:
  Constant1/1 -> AyDtLimit/1

== matlab function PvtSubSys_LATC/LATC/LateralControl/MATLAB Function ==
  data: desLaneA0 input; FLg output; desLaneA1 input; A0_Limit input; A1_Limit input
function FLg = fcn(desLaneA0,desLaneA1,A0_Limit,A1_Limit)
FLg = uint8(0);
if (desLaneA0<A0_Limit)&&(desLaneA1<A1_Limit) %可以激活换道和完成换道
    FLg = uint8(1);
end
end

== matlab function PvtSubSys_LATC/LATC/LateralControl/LCS_Angle/Controller/StateErrorCalc/MATLAB Function ==
  data: Lookahead_Distance input; Ego_X input; Ego_Y input; Traj_X input; Traj_Y input; Traj_Heading input; Traj_Kappa input; Traj_S input; lookahead_Pt_X output; Target_Pt_X input; Target_Pt_Y input; Target_Pt_S input; lookahead_Pt_Y output; lookahead_Pt_Heading output; lookahead_Pt_Kappa output single; Lookahead_Pt_Num output
%% 为横向控制找预瞄点
function [lookahead_Pt_X,lookahead_Pt_Y,lookahead_Pt_Heading,lookahead_Pt_Kappa,Lookahead_Pt_Num]= ...
QueryLookaheadPointByPosition(Lookahead_Distance,Ego_X,Ego_Y,Traj_X,Traj_Y,Traj_Heading,Traj_Kappa,Traj_S,Target_Pt_X,Target_Pt_Y,Target_Pt_S)

    target_dist=((Target_Pt_X-Ego_X)^2+((Target_Pt_Y-Ego_Y)^2))^0.5;
    % lookahead_index=0;
    for i=1:length(Traj_X)
        %找到轨迹上累积弧长之差超过此距离的点作为预瞄点 
        %到目标点距离，再加上第i个点与目标点的弧长s之差刚好大于预瞄距离的那个点
        lookahead_dist = Traj_S(i,1)-Target_Pt_S(1,1)+target_dist;
        
        if(lookahead_dist>=Lookahead_Distance)
            lookahead_index = i;
            lookahead_Pt_X= Traj_X(lookahead_index,1);
            lookahead_Pt_Y= Traj_Y(lookahead_index,1);
            lookahead_Pt_Heading= Traj_Heading(lookahead_index,1);
            lookahead_Pt_Kappa= Traj_Kappa(lookahead_index,1);
            Lookahead_Pt_Num = i;
            return
        end
        %若遍历到最后一个点也没有大于lookahead_station的就取最后一个点
        lookahead_Pt_X= Traj_X(i,1);
        lookahead_Pt_Y= Traj_Y(i,1);
        lookahead_Pt_Heading= Traj_Heading(i,1);
        lookahead_Pt_Kappa= Traj_Kappa(i,1);
    end
    Lookahead_Pt_Num = i;
end

== matlab function PvtSubSys_LATC/communicationTest3/MATLAB Function7 ==
  data: factor input single; singlemin input single; singlemax input single; singleoutK1 input single; singleout output single; countk1 input uint8; count output uint8
function [singleout,count] = single(factor,singlemin,singlemax,singleoutK1,countk1)
count=countk1+uint8(1);
singleout=singleoutK1;
if count>=100
    count=uint8(0);
end
if count==99
    singleout=singleoutK1+factor;
    if singleout>singlemax
        singleout=singlemin;
    end      
end

== matlab function PvtSubSys_LATC/communicationTest1/MATLAB Function19 ==
  data: uint8outK1 input uint8; uint8out output uint8; countk1 input uint8; count output uint8
function [uint8out,count] = uint8(uint8outK1,countk1)
count=countk1+uint8(1);
uint8out=uint8outK1;
if count>=100
    count=uint8(0);
end
if count==99
    uint8out=uint8outK1+uint8(1);
    if uint8out>2
        uint8out=uint8(0);
    end      
end

== matlab function PvtSubSys_LATC/LATC/LateralControl/LCS_Angle/Trajectory_Points/RoadCreate/Subsystem/MATLAB Function1 ==
  data: Delaytime input uint16; Flg output uint8; Count output uint16; TarDangerLevel input uint8; TarDangerLevelK1 input uint8; FlgK1 input uint8; CountK1 input uint16
function [Flg,Count]= fcn(Delaytime,TarDangerLevel,TarDangerLevelK1,FlgK1,CountK1)
Count = min(CountK1 + uint16(1),Delaytime);
if Count == Delaytime
    Flg = uint8(0);
else
    Flg = FlgK1;
end
%%状态检测
if TarDangerLevel == uint8(1) && TarDangerLevelK1 == 1 %功能激活
    Count = uint16(0);
    Flg = uint8(1);  
end
if  TarDangerLevel==uint8(3) && (TarDangerLevelK1==uint8(1)||TarDangerLevelK1==uint8(2)) % LCK/IE 2 LC_Normal
    Count =uint16(0);
    Flg = uint8(2);
end

if  TarDangerLevel==uint8(7) && (TarDangerLevelK1==uint8(1)||TarDangerLevelK1==uint8(2)) % LCK/IE 2 LC_Eco
    Count =uint16(0);
    Flg = uint8(3);
end

if  TarDangerLevel==uint8(8) && (TarDangerLevelK1==uint8(1)||TarDangerLevelK1==uint8(2)) % LCK/IE 2 LC_sport
    Count =uint16(0);
    Flg = uint8(4);
end
end

== matlab function PvtSubSys_LATC/communicationTest4/MATLAB Function7 ==
  data: factor input single; singlemin input single; singlemax input single; singleoutK1 input single; singleout output single; countk1 input uint8; count output uint8
function [singleout,count] = single(factor,singlemin,singlemax,singleoutK1,countk1)
count=countk1+uint8(1);
singleout=singleoutK1;
if count>=100
    count=uint8(0);
end
if count==99
    singleout=singleoutK1+factor;
    if singleout>singlemax
        singleout=singlemin;
    end      
end
